simulink model "filter_taua"  (R2022a)
settings: Solver=ode1  StartTime=0.0  StopTime=100  FixedStep=Ts  RelTol=1e-3
undefined symbols (not defined in the file or in its folder): tau_A, tau_C, tau_D
settings Model: Creator=stt  LastModifiedBy=stt

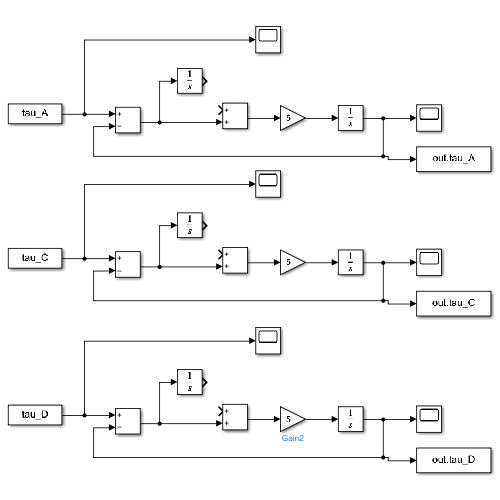
[thumbnail: Simulink's stored preview of the top-level diagram]
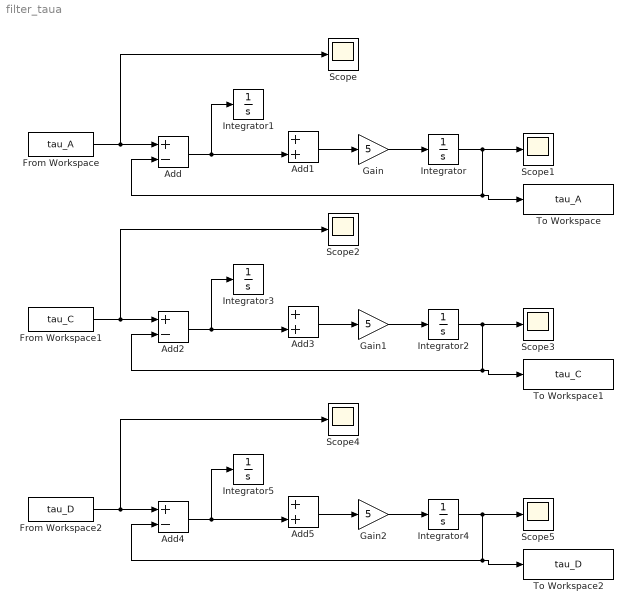
== system filter_taua ==
  Add : Sum  Inputs=+-
  Add1 : Sum
  Add2 : Sum  Inputs=+-
  Add3 : Sum
  Add4 : Sum  Inputs=+-
  Add5 : Sum
  From Workspace : FromWorkspace  VariableName=tau_A
  From Workspace1 : FromWorkspace  VariableName=tau_C
  From Workspace2 : FromWorkspace  VariableName=tau_D
  Gain : Gain  Gain=5
  Gain1 : Gain  Gain=5
  Gain2 : Gain  Gain=5
  Integrator : Integrator  InitialCondition=tau_A.signals.values(1)
  Integrator1 : Integrator
  Integrator2 : Integrator  InitialCondition=tau_C.signals.values(1)
  Integrator3 : Integrator
  Integrator4 : Integrator  InitialCondition=tau_D.signals.values(1)
  Integrator5 : Integrator
  Scope{,1..5} (6 alike) : Scope
  To Workspace : ToWorkspace  VariableName=tau_A  SampleTime=-1
  To Workspace1 : ToWorkspace  VariableName=tau_C  SampleTime=-1
  To Workspace2 : ToWorkspace  VariableName=tau_D  SampleTime=-1
  wires:
  Gain/1 -> Integrator/1
  Add/1 -> Add1/2, Integrator1/1
  Add1/1 -> Gain/1
  Integrator/1 -> Scope1/1, To Workspace/1, Add/2
  From Workspace/1 -> Scope/1, Add/1
  Add2/1 -> Add3/2, Integrator3/1
  Add3/1 -> Gain1/1
  Gain1/1 -> Integrator2/1
  Integrator2/1 -> Scope3/1, To Workspace1/1, Add2/2
  From Workspace1/1 -> Scope2/1, Add2/1
  Add4/1 -> Add5/2, Integrator5/1
  Add5/1 -> Gain2/1
  Gain2/1 -> Integrator4/1
  Integrator4/1 -> Scope5/1, To Workspace2/1, Add4/2
  From Workspace2/1 -> Scope4/1, Add4/1
